simulink model "EHB_speedgoat_R2020a_V1"  (R2020a)
settings: Solver=FixedStepDiscrete  StartTime=0.0  StopTime=inf  FixedStep=0.001  RelTol=1e-3  EnableMultiTasking=on
model workspace (MAT data in the model file):
  A : Simulink.Signal (value not decoded)
  B : Simulink.Signal (value not decoded)
  C : Simulink.Signal (value not decoded)
  D : Simulink.Signal (value not decoded)
  E : Simulink.Signal (value not decoded)
  calin = [-9.96 -7.98 -5.98 -3.99 -1.994 0 1.995 3.992 5.99 7.98 9.97]
  calout = [-10 -8 -6 -4 -2 0 2 4 6 8 10]
symbols that are objects in the model workspace (value not decoded): C, D
undefined symbols (not defined in the file): Com1, none, ts_IO612
libraries: simulink x1436, xpcethercatlib x1223, yisutbxlib_utilities x256, xpcutilitieslib x156, hdlsllib x145, canmsglib x46, speedgoatlib_IO602_4 x11, speedgoatlib_IO611 x7, slrttcplib x4, CanManageLib x3, slrtlib x3, xpcseriallib x2
(part 10 of 30)

== system EHB_speedgoat_R2020a_V1/保留/TIF_06/CB1032_2/PWM ==
  Display{,1..63} (64 alike) : Display
  PCAP_DUTY_{1..32} (32 alike) : Gain
  PCAP_PER_{1..32} (32 alike) : Gain
  PWMCAP1 : Subsystem  mask(simucat_pwmcap){deviceID=0, boxNum=Box 2 (Digital Board), channel1=on, channel2=on, channel3=on, channel4=on, channel5=on, channel6=on, channel7=on, channel8=on, channel9=on, channel10=on, channel11=on, channel12=on, channel13=on, channel14=on, channel15=on, channel16=on, channel17=on, channel18=on, channel19=on, channel20=on, channel21=on, channel22=on, channel23=on, channel24=on, channel25=on, channel26=on, channel27=on, channel28=on, channel29=on, channel30=on, channel31=on, channel32=on, capMode=automatic}
      mask prompts: deviceID "Device Index:"; boxNum "Select a box:"; channel1 "1"; channel2 "2"; channel3 "3"; channel4 "4"; channel5 "5"; channel6 "6"; channel7 "7"; channel8 "8"; channel9 "9"; channel10 "10"; channel11 "11"; channel12 "12"; channel13 "13"; channel14 "14"; channel15 "15"; channel16 "16"; channel17 "17"; channel18 "18"; channel19 "19"; channel20 "20"; channel21 "21"; channel22 "22"; channel23 "23"; channel24 "24"; channel25 "25"; channel26 "26"; channel27 "27"; channel28 "28"; channel29 "29"; channel30 "30"; channel31 "31"; channel32 "32"; capMode "Cap Mode"
      mask help:
      | SimuCat系列数字板卡驱动模块。
      | 功能：PWM波捕获。通道数：32
      mask TypeOptions deviceID: 0 | 1 | 2 | 3 | 4 | 5 | 6 | 7 | 8 | 9 | 10 | 11 | 12 | 13 | 14 | 15
      mask TypeOptions boxNum: Box 1 (Digital Board) | Box 2 (Digital Board) | Box 3 (Digital Board) | Box 4 (Digital Board)
      mask TypeOptions capMode: automatic | manual
      mask DialogControl refreshButton Prompt: Refresh
      mask DialogControl refreshButton Callback: ystbx.mask.callbacks.refreshBoxList
      mask DialogControl selectChannel Prompt: Select channels:
      mask DialogControl Dummy Prompt: (Add text here)
      mask DialogControl channelSelectAll Prompt: Select All
      mask DialogControl channelSelectAll Callback: ystbx.mask.callbacks.selectAllChannels();
      mask DialogControl channelClearAll Prompt: Clear All
      mask DialogControl channelClearAll Callback: ystbx.mask.callbacks.clearAllChannels();
      mask DialogControl applyButton Prompt: Apply Modification
      mask DialogControl applyButton Callback: ystbx.mask.callbacks.maskApply();
      mask Display: disp('CB1032(Digital Board)\nPWM signal capture\nNetwork Device 0\nBox 2 (Digital Board)');port_label('output',1,'PWMCAP_DutyCycle_CH1');port_label('output',2,'PWMCAP_Period_CH1');port_label('output',3,'PWMCAP_DutyCycle_CH2');port_label('output',4,'PWMCAP_Period_CH2');port_label('output',5,'PWMCAP_DutyCycle_CH3');port_label('output',6,'PWMCAP_Period_CH3');port_label('output',7,'PWMCAP_DutyCycle_CH4');port_label('output',8,'PWMCAP_Period_CH4');port_label('output',9,'PWMCAP_DutyCycle_CH5');port_label('output',10,'PWMCAP_Period_CH5');port_label('output',11,'PWMCAP_DutyCycle_CH6');port_label('output',12,'PWMCAP_Period_CH6');port_label('output',13,'PWMCAP_DutyCycle_CH7');port_label('output',14,'PWMCAP_Period_CH7');port_label('output',15,'PWMCAP_DutyCycle_CH8');port_label('output',16,'PWMCAP_Period_CH8');port_label('output',17,'PWMCAP_DutyCycle_CH9');port_label('output',18,'PWMCAP_Period_CH9');port_label('output',19,'PWMCAP_DutyCycle_CH10');port_label('output',20,'PWMCAP_Period_CH10');port_label('output',21,'PWMCAP_DutyCycle_CH11');port_label('output',22,'PWMCAP_Period_CH11');port_label('output',23,'PWMCAP_DutyCycle_CH12');port_label('output',24,'PWMCAP_Period_CH12');port_label('output',25,'PWMCAP_DutyCycle_CH13');port_label('output',26,'PWMCAP_Period_CH13');port_label('output',27,'PWMCAP_DutyCycle_CH14');port_label('output',28,'PWMCAP_Period_CH14');port_label('output',29,'PWMCAP_DutyCycle_CH15');port_label('output',30,'PWMCAP_Period_CH15');port_label('output',31,'PWMCAP_DutyCycle_CH16');port_label('output',32,'PWMCAP_Period_CH16');port_label('output',33,'PWMCAP_DutyCycle_CH17');port_label('output',34,'PWMCAP_Period_CH17');port_label('output',35,'PWMCAP_DutyCycle_CH18');port_label('output',36,'PWMCAP_Period_CH18');port_label('output',37,'PWMCAP_DutyCycle_CH19');port_label('output',38,'PWMCAP_Period_CH19');port_label('output',39,'PWMCAP_DutyCycle_CH20');port_label('output',40,'PWMCAP_Period_CH20');port_label('output',41,'PWMCAP_DutyCycle_CH21');port_label('output',42,'PWMCAP_Period_CH21');port_label('output',43,'PWMCAP_DutyCycle_CH22');port_label('output',44,'PWMCAP_Period_CH22');port_label('output',45,'PWMCAP_DutyCycle_CH23');port_label('output',46,'PWMCAP_Period_CH23');port_label('output',47,'PWMCAP_DutyCycle_CH24');port_label('output',48,'PWMCAP_Period_CH24');port_label('output',49,'PWMCAP_DutyCycle_CH25');port_label('output',50,'PWMCAP_Period_CH25');port_label('output',51,'PWMCAP_DutyCycle_CH26');port_label('output',52,'PWMCAP_Period_CH26');port_label('output',53,'PWMCAP_DutyCycle_CH27');port_label('output',54,'PWMCAP_Period_CH27');port_label('output',55,'PWMCAP_DutyCycle_CH28');port_label('output',56,'PWMCAP_Period_CH28');port_label('output',57,'PWMCAP_DutyCycle_CH29');port_label('output',58,'PWMCAP_Period_CH29');port_label('output',59,'PWMCAP_DutyCycle_CH30');port_label('output',60,'PWMCAP_Period_CH30');port_label('output',61,'PWMCAP_DutyCycle_CH31');port_label('output',62,'PWMCAP_Period_CH31');port_label('output',63,'PWMCAP_DutyCycle_CH32');port_label('output',64,'PWMCAP_Period_CH32');
  PWMOUT : Subsystem  mask(simucat_pwmout){deviceID=0, boxNum=Box 2 (Digital Board), channel1=on, channel2=on, channel3=on, channel4=on, channel5=on, channel6=on, channel7=on, channel8=on, channel9=on, channel10=on, channel11=on, channel12=on, channel13=on, channel14=on, channel15=on, channel16=on, channel17=on, channel18=on, channel19=on, channel20=on, channel21=on, channel22=on, channel23=on, channel24=on, channel25=on, channel26=on, channel27=on, channel28=on, channel29=on, channel30=on, channel31=on, channel32=on}
      mask prompts: deviceID "Device Index:"; boxNum "Select a box:"; channel1 "1"; channel2 "2"; channel3 "3"; channel4 "4"; channel5 "5"; channel6 "6"; channel7 "7"; channel8 "8"; channel9 "9"; channel10 "10"; channel11 "11"; channel12 "12"; channel13 "13"; channel14 "14"; channel15 "15"; channel16 "16"; channel17 "17"; channel18 "18"; channel19 "19"; channel20 "20"; channel21 "21"; channel22 "22"; channel23 "23"; channel24 "24"; channel25 "25"; channel26 "26"; channel27 "27"; channel28 "28"; channel29 "29"; channel30 "30"; channel31 "31"; channel32 "32"
      mask help:
      | SimuCat系列数字板卡驱动模块。
      | 功能：PWM波输出。通道数：32
      mask TypeOptions deviceID: 0 | 1 | 2 | 3 | 4 | 5 | 6 | 7 | 8 | 9 | 10 | 11 | 12 | 13 | 14 | 15
      mask TypeOptions boxNum: Box 1 (Digital Board) | Box 2 (Digital Board) | Box 3 (Digital Board) | Box 4 (Digital Board)
      mask DialogControl refreshButton Prompt: Refresh
      mask DialogControl refreshButton Callback: ystbx.mask.callbacks.refreshBoxList
      mask DialogControl selectChannel Prompt: Select channels:
      mask DialogControl Dummy Prompt: (Add text here)
      mask DialogControl channelSelectAll Prompt: Select All
      mask DialogControl channelSelectAll Callback: ystbx.mask.callbacks.selectAllChannels();
      mask DialogControl channelClearAll Prompt: Clear All
      mask DialogControl channelClearAll Callback: ystbx.mask.callbacks.clearAllChannels();
      mask DialogControl applyButton Prompt: Apply Modification
      mask DialogControl applyButton Callback: ystbx.mask.callbacks.maskApply();
      mask Display: disp('CB1032(Digital Board)\nPWM signal output\nNetwork Device 0\nBox 2 (Digital Board)');port_label('input',1,'PWMOUT_DutyCycle_CH1');port_label('input',2,'PWMOUT_Period_CH1');port_label('input',3,'PWMOUT_DutyCycle_CH2');port_label('input',4,'PWMOUT_Period_CH2');port_label('input',5,'PWMOUT_DutyCycle_CH3');port_label('input',6,'PWMOUT_Period_CH3');port_label('input',7,'PWMOUT_DutyCycle_CH4');port_label('input',8,'PWMOUT_Period_CH4');port_label('input',9,'PWMOUT_DutyCycle_CH5');port_label('input',10,'PWMOUT_Period_CH5');port_label('input',11,'PWMOUT_DutyCycle_CH6');port_label('input',12,'PWMOUT_Period_CH6');port_label('input',13,'PWMOUT_DutyCycle_CH7');port_label('input',14,'PWMOUT_Period_CH7');port_label('input',15,'PWMOUT_DutyCycle_CH8');port_label('input',16,'PWMOUT_Period_CH8');port_label('input',17,'PWMOUT_DutyCycle_CH9');port_label('input',18,'PWMOUT_Period_CH9');port_label('input',19,'PWMOUT_DutyCycle_CH10');port_label('input',20,'PWMOUT_Period_CH10');port_label('input',21,'PWMOUT_DutyCycle_CH11');port_label('input',22,'PWMOUT_Period_CH11');port_label('input',23,'PWMOUT_DutyCycle_CH12');port_label('input',24,'PWMOUT_Period_CH12');port_label('input',25,'PWMOUT_DutyCycle_CH13');port_label('input',26,'PWMOUT_Period_CH13');port_label('input',27,'PWMOUT_DutyCycle_CH14');port_label('input',28,'PWMOUT_Period_CH14');port_label('input',29,'PWMOUT_DutyCycle_CH15');port_label('input',30,'PWMOUT_Period_CH15');port_label('input',31,'PWMOUT_DutyCycle_CH16');port_label('input',32,'PWMOUT_Period_CH16');port_label('input',33,'PWMOUT_DutyCycle_CH17');port_label('input',34,'PWMOUT_Period_CH17');port_label('input',35,'PWMOUT_DutyCycle_CH18');port_label('input',36,'PWMOUT_Period_CH18');port_label('input',37,'PWMOUT_DutyCycle_CH19');port_label('input',38,'PWMOUT_Period_CH19');port_label('input',39,'PWMOUT_DutyCycle_CH20');port_label('input',40,'PWMOUT_Period_CH20');port_label('input',41,'PWMOUT_DutyCycle_CH21');port_label('input',42,'PWMOUT_Period_CH21');port_label('input',43,'PWMOUT_DutyCycle_CH22');port_label('input',44,'PWMOUT_Period_CH22');port_label('input',45,'PWMOUT_DutyCycle_CH23');port_label('input',46,'PWMOUT_Period_CH23');port_label('input',47,'PWMOUT_DutyCycle_CH24');port_label('input',48,'PWMOUT_Period_CH24');port_label('input',49,'PWMOUT_DutyCycle_CH25');port_label('input',50,'PWMOUT_Period_CH25');port_label('input',51,'PWMOUT_DutyCycle_CH26');port_label('input',52,'PWMOUT_Period_CH26');port_label('input',53,'PWMOUT_DutyCycle_CH27');port_label('input',54,'PWMOUT_Period_CH27');port_label('input',55,'PWMOUT_DutyCycle_CH28');port_label('input',56,'PWMOUT_Period_CH28');port_label('input',57,'PWMOUT_DutyCycle_CH29');port_label('input',58,'PWMOUT_Period_CH29');port_label('input',59,'PWMOUT_DutyCycle_CH30');port_label('input',60,'PWMOUT_Period_CH30');port_label('input',61,'PWMOUT_DutyCycle_CH31');port_label('input',62,'PWMOUT_Period_CH31');port_label('input',63,'PWMOUT_DutyCycle_CH32');port_label('input',64,'PWMOUT_Period_CH32');
  PoDu_CH1 : Constant  Value=0.7
  PoDu_CH{2..32} (31 alike) : Constant  Value=0.5
  PoPe_CH{1..32} (32 alike) : Constant  Value=1/20000
  wires:
  PCAP_DUTY_30/1 -> Display58/1  "PCAP_DUTY_30"
  PCAP_DUTY_1/1 -> Display/1  "PCAP_DUTY_1"
  PCAP_DUTY_15/1 -> Display36/1  "PCAP_DUTY_15"
  PCAP_DUTY_13/1 -> Display46/1  "PCAP_DUTY_13"
  PCAP_PER_3/1 -> Display5/1  "PCAP_PER_3"
  PCAP_DUTY_19/1 -> Display20/1  "PCAP_DUTY_19"
  PCAP_DUTY_31/1 -> Display60/1  "PCAP_DUTY_31"
  PCAP_DUTY_27/1 -> Display52/1  "PCAP_DUTY_27"
  PCAP_PER_18/1 -> Display19/1  "PCAP_PER_18"
  PCAP_DUTY_32/1 -> Display62/1  "PCAP_DUTY_32"
  PCAP_DUTY_25/1 -> Display48/1  "PCAP_DUTY_25"
  PCAP_DUTY_17/1 -> Display16/1  "PCAP_DUTY_17"
  PCAP_PER_6/1 -> Display11/1  "PCAP_PER_6"
  PCAP_PER_15/1 -> Display37/1  "PCAP_PER_15"
  PCAP_PER_2/1 -> Display3/1  "PCAP_PER_2"
  PCAP_DUTY_6/1 -> Display10/1  "PCAP_DUTY_6"
  PCAP_PER_4/1 -> Display7/1  "PCAP_PER_4"
  PCAP_PER_17/1 -> Display17/1  "PCAP_PER_17"
  PCAP_DUTY_18/1 -> Display18/1  "PCAP_DUTY_18"
  PCAP_DUTY_21/1 -> Display24/1  "PCAP_DUTY_21"
  PCAP_PER_12/1 -> Display45/1  "PCAP_PER_12"
  PCAP_DUTY_10/1 -> Display40/1  "PCAP_DUTY_10"
  PCAP_PER_23/1 -> Display29/1  "PCAP_PER_23"
  PCAP_DUTY_26/1 -> Display50/1  "PCAP_DUTY_26"
  PCAP_DUTY_20/1 -> Display22/1  "PCAP_DUTY_20"
  PCAP_PER_19/1 -> Display21/1  "PCAP_PER_19"
  PCAP_DUTY_12/1 -> Display44/1  "PCAP_DUTY_12"
  PCAP_PER_29/1 -> Display57/1  "PCAP_PER_29"
  PCAP_PER_21/1 -> Display25/1  "PCAP_PER_21"
  PCAP_PER_1/1 -> Display1/1  "PCAP_PER_1"
  PCAP_DUTY_29/1 -> Display56/1  "PCAP_DUTY_29"
  PCAP_DUTY_2/1 -> Display2/1  "PCAP_DUTY_2"
  PCAP_PER_27/1 -> Display53/1  "PCAP_PER_27"
  PCAP_PER_8/1 -> Display15/1  "PCAP_PER_8"
  PCAP_PER_7/1 -> Display13/1  "PCAP_PER_7"
  PCAP_DUTY_7/1 -> Display12/1  "PCAP_DUTY_7"
  PCAP_DUTY_8/1 -> Display14/1  "PCAP_DUTY_8"
  PCAP_PER_24/1 -> Display31/1  "PCAP_PER_24"
  PCAP_PER_22/1 -> Display27/1  "PCAP_PER_22"
  PCAP_DUTY_28/1 -> Display54/1  "PCAP_DUTY_28"
  PCAP_PER_16/1 -> Display39/1  "PCAP_PER_16"
  PCAP_DUTY_11/1 -> Display42/1  "PCAP_DUTY_11"
  PCAP_DUTY_24/1 -> Display30/1  "PCAP_DUTY_24"
  PCAP_PER_30/1 -> Display59/1  "PCAP_PER_30"
  PCAP_DUTY_16/1 -> Display38/1  "PCAP_DUTY_16"
  PCAP_DUTY_4/1 -> Display6/1  "PCAP_DUTY_4"
  PCAP_DUTY_14/1 -> Display34/1  "PCAP_DUTY_14"
  PCAP_PER_10/1 -> Display41/1  "PCAP_PER_10"
  PCAP_PER_20/1 -> Display23/1  "PCAP_PER_20"
  PCAP_PER_26/1 -> Display51/1  "PCAP_PER_26"
  PCAP_PER_32/1 -> Display63/1  "PCAP_PER_32"
  PCAP_DUTY_5/1 -> Display8/1  "PCAP_DUTY_5"
  PCAP_DUTY_3/1 -> Display4/1  "PCAP_DUTY_3"
  PCAP_PER_5/1 -> Display9/1  "PCAP_PER_5"
  PCAP_DUTY_23/1 -> Display28/1  "PCAP_DUTY_23"
  PCAP_DUTY_22/1 -> Display26/1  "PCAP_DUTY_22"
  PCAP_DUTY_9/1 -> Display32/1  "PCAP_DUTY_9"
  PCAP_PER_25/1 -> Display49/1  "PCAP_PER_25"
  PCAP_PER_13/1 -> Display47/1  "PCAP_PER_13"
  PCAP_PER_9/1 -> Display33/1  "PCAP_PER_9"
  PCAP_PER_28/1 -> Display55/1  "PCAP_PER_28"
  PCAP_PER_31/1 -> Display61/1  "PCAP_PER_31"
  PCAP_PER_11/1 -> Display43/1  "PCAP_PER_11"
  PCAP_PER_14/1 -> Display35/1  "PCAP_PER_14"
  PWMCAP1/2(PWMCAP_Period_CH1) -> PCAP_PER_1/1
  PWMCAP1/4(PWMCAP_Period_CH2) -> PCAP_PER_2/1
  PWMCAP1/6(PWMCAP_Period_CH3) -> PCAP_PER_3/1
  PWMCAP1/8(PWMCAP_Period_CH4) -> PCAP_PER_4/1
  PWMCAP1/10(PWMCAP_Period_CH5) -> PCAP_PER_5/1
  PWMCAP1/12(PWMCAP_Period_CH6) -> PCAP_PER_6/1
  PWMCAP1/14(PWMCAP_Period_CH7) -> PCAP_PER_7/1
  PWMCAP1/16(PWMCAP_Period_CH8) -> PCAP_PER_8/1
  PWMCAP1/18(PWMCAP_Period_CH9) -> PCAP_PER_9/1
  PWMCAP1/20(PWMCAP_Period_CH10) -> PCAP_PER_10/1
  PWMCAP1/22(PWMCAP_Period_CH11) -> PCAP_PER_11/1
  PWMCAP1/24(PWMCAP_Period_CH12) -> PCAP_PER_12/1
  PWMCAP1/26(PWMCAP_Period_CH13) -> PCAP_PER_13/1
  PWMCAP1/28(PWMCAP_Period_CH14) -> PCAP_PER_14/1
  PWMCAP1/30(PWMCAP_Period_CH15) -> PCAP_PER_15/1
  PWMCAP1/32(PWMCAP_Period_CH16) -> PCAP_PER_16/1
  PWMCAP1/34(PWMCAP_Period_CH17) -> PCAP_PER_17/1
  PWMCAP1/36(PWMCAP_Period_CH18) -> PCAP_PER_18/1
  PWMCAP1/38(PWMCAP_Period_CH19) -> PCAP_PER_19/1
  PWMCAP1/40(PWMCAP_Period_CH20) -> PCAP_PER_20/1
  PWMCAP1/42(PWMCAP_Period_CH21) -> PCAP_PER_21/1
  PWMCAP1/44(PWMCAP_Period_CH22) -> PCAP_PER_22/1
  PWMCAP1/46(PWMCAP_Period_CH23) -> PCAP_PER_23/1
  PWMCAP1/48(PWMCAP_Period_CH24) -> PCAP_PER_24/1
  PWMCAP1/50(PWMCAP_Period_CH25) -> PCAP_PER_25/1
  PWMCAP1/52(PWMCAP_Period_CH26) -> PCAP_PER_26/1
  PWMCAP1/54(PWMCAP_Period_CH27) -> PCAP_PER_27/1
  PWMCAP1/56(PWMCAP_Period_CH28) -> PCAP_PER_28/1
  PWMCAP1/58(PWMCAP_Period_CH29) -> PCAP_PER_29/1
  PWMCAP1/60(PWMCAP_Period_CH30) -> PCAP_PER_30/1
  PWMCAP1/62(PWMCAP_Period_CH31) -> PCAP_PER_31/1
  PWMCAP1/64(PWMCAP_Period_CH32) -> PCAP_PER_32/1
  PWMCAP1/1(PWMCAP_DutyCycle_CH1) -> PCAP_DUTY_1/1
  PWMCAP1/3(PWMCAP_DutyCycle_CH2) -> PCAP_DUTY_2/1
  PWMCAP1/5(PWMCAP_DutyCycle_CH3) -> PCAP_DUTY_3/1
  PWMCAP1/7(PWMCAP_DutyCycle_CH4) -> PCAP_DUTY_4/1
  PWMCAP1/9(PWMCAP_DutyCycle_CH5) -> PCAP_DUTY_5/1
  PWMCAP1/11(PWMCAP_DutyCycle_CH6) -> PCAP_DUTY_6/1
  PWMCAP1/13(PWMCAP_DutyCycle_CH7) -> PCAP_DUTY_7/1
  PWMCAP1/15(PWMCAP_DutyCycle_CH8) -> PCAP_DUTY_8/1
  PWMCAP1/17(PWMCAP_DutyCycle_CH9) -> PCAP_DUTY_9/1
  PWMCAP1/19(PWMCAP_DutyCycle_CH10) -> PCAP_DUTY_10/1
  PWMCAP1/21(PWMCAP_DutyCycle_CH11) -> PCAP_DUTY_11/1
  PWMCAP1/23(PWMCAP_DutyCycle_CH12) -> PCAP_DUTY_12/1
  PWMCAP1/25(PWMCAP_DutyCycle_CH13) -> PCAP_DUTY_13/1
  PWMCAP1/27(PWMCAP_DutyCycle_CH14) -> PCAP_DUTY_14/1
  PWMCAP1/29(PWMCAP_DutyCycle_CH15) -> PCAP_DUTY_15/1
  PWMCAP1/31(PWMCAP_DutyCycle_CH16) -> PCAP_DUTY_16/1
  PWMCAP1/33(PWMCAP_DutyCycle_CH17) -> PCAP_DUTY_17/1
  PWMCAP1/35(PWMCAP_DutyCycle_CH18) -> PCAP_DUTY_18/1
  PWMCAP1/37(PWMCAP_DutyCycle_CH19) -> PCAP_DUTY_19/1
  PWMCAP1/39(PWMCAP_DutyCycle_CH20) -> PCAP_DUTY_20/1
  PWMCAP1/41(PWMCAP_DutyCycle_CH21) -> PCAP_DUTY_21/1
  PWMCAP1/43(PWMCAP_DutyCycle_CH22) -> PCAP_DUTY_22/1
  PWMCAP1/45(PWMCAP_DutyCycle_CH23) -> PCAP_DUTY_23/1
  PWMCAP1/47(PWMCAP_DutyCycle_CH24) -> PCAP_DUTY_24/1
  PWMCAP1/49(PWMCAP_DutyCycle_CH25) -> PCAP_DUTY_25/1
  PWMCAP1/51(PWMCAP_DutyCycle_CH26) -> PCAP_DUTY_26/1
  PWMCAP1/53(PWMCAP_DutyCycle_CH27) -> PCAP_DUTY_27/1
  PWMCAP1/55(PWMCAP_DutyCycle_CH28) -> PCAP_DUTY_28/1
  PWMCAP1/57(PWMCAP_DutyCycle_CH29) -> PCAP_DUTY_29/1
  PWMCAP1/59(PWMCAP_DutyCycle_CH30) -> PCAP_DUTY_30/1
  PWMCAP1/61(PWMCAP_DutyCycle_CH31) -> PCAP_DUTY_31/1
  PWMCAP1/63(PWMCAP_DutyCycle_CH32) -> PCAP_DUTY_32/1
  PoDu_CH19/1 -> PWMOUT/37(PWMOUT_DutyCycle_CH19)  "PoDu_CH19"
  PoPe_CH19/1 -> PWMOUT/38(PWMOUT_Period_CH19)  "PoPe_CH19"
  PoDu_CH20/1 -> PWMOUT/39(PWMOUT_DutyCycle_CH20)  "PoDu_CH20"
  PoPe_CH21/1 -> PWMOUT/42(PWMOUT_Period_CH21)  "PoPe_CH21"
  PoDu_CH22/1 -> PWMOUT/43(PWMOUT_DutyCycle_CH22)  "PoDu_CH22"
  PoDu_CH1/1 -> PWMOUT/1(PWMOUT_DutyCycle_CH1)  "PoDu_CH17"
  PoPe_CH1/1 -> PWMOUT/2(PWMOUT_Period_CH1)  "PoPe_CH17"
  PoDu_CH2/1 -> PWMOUT/3(PWMOUT_DutyCycle_CH2)  "PoDu_CH18"
  PoPe_CH2/1 -> PWMOUT/4(PWMOUT_Period_CH2)  "PoPe_CH18"
  PoDu_CH3/1 -> PWMOUT/5(PWMOUT_DutyCycle_CH3)  "PoDu_CH19"
  PoPe_CH3/1 -> PWMOUT/6(PWMOUT_Period_CH3)  "PoPe_CH19"
  PoDu_CH4/1 -> PWMOUT/7(PWMOUT_DutyCycle_CH4)  "PoDu_CH20"
  PoPe_CH4/1 -> PWMOUT/8(PWMOUT_Period_CH4)  "PoPe_CH20"
  PoDu_CH5/1 -> PWMOUT/9(PWMOUT_DutyCycle_CH5)  "PoDu_CH21"
  PoPe_CH5/1 -> PWMOUT/10(PWMOUT_Period_CH5)  "PoPe_CH21"
  PoDu_CH6/1 -> PWMOUT/11(PWMOUT_DutyCycle_CH6)  "PoDu_CH22"
  PoPe_CH6/1 -> PWMOUT/12(PWMOUT_Period_CH6)  "PoPe_CH22"
  PoDu_CH7/1 -> PWMOUT/13(PWMOUT_DutyCycle_CH7)  "PoDu_CH23"
  PoPe_CH7/1 -> PWMOUT/14(PWMOUT_Period_CH7)  "PoPe_CH23"
  PoDu_CH8/1 -> PWMOUT/15(PWMOUT_DutyCycle_CH8)  "PoDu_CH24"
  PoPe_CH8/1 -> PWMOUT/16(PWMOUT_Period_CH8)  "PoPe_CH24"
  PoDu_CH9/1 -> PWMOUT/17(PWMOUT_DutyCycle_CH9)  "PoDu_CH25"
  PoPe_CH9/1 -> PWMOUT/18(PWMOUT_Period_CH9)  "PoPe_CH25"
  PoDu_CH10/1 -> PWMOUT/19(PWMOUT_DutyCycle_CH10)  "PoDu_CH26"
  PoPe_CH10/1 -> PWMOUT/20(PWMOUT_Period_CH10)  "PoPe_CH26"
  PoDu_CH11/1 -> PWMOUT/21(PWMOUT_DutyCycle_CH11)  "PoDu_CH27"
  PoPe_CH11/1 -> PWMOUT/22(PWMOUT_Period_CH11)  "PoPe_CH27"
  PoDu_CH12/1 -> PWMOUT/23(PWMOUT_DutyCycle_CH12)  "PoDu_CH28"
  PoPe_CH12/1 -> PWMOUT/24(PWMOUT_Period_CH12)  "PoPe_CH28"
  PoDu_CH13/1 -> PWMOUT/25(PWMOUT_DutyCycle_CH13)  "PoDu_CH29"
  PoPe_CH13/1 -> PWMOUT/26(PWMOUT_Period_CH13)  "PoPe_CH29"
  PoDu_CH14/1 -> PWMOUT/27(PWMOUT_DutyCycle_CH14)  "PoDu_CH30"
  PoPe_CH14/1 -> PWMOUT/28(PWMOUT_Period_CH14)  "PoPe_CH30"
  PoDu_CH15/1 -> PWMOUT/29(PWMOUT_DutyCycle_CH15)  "PoDu_CH31"
  PoPe_CH15/1 -> PWMOUT/30(PWMOUT_Period_CH15)  "PoPe_CH31"
  PoDu_CH16/1 -> PWMOUT/31(PWMOUT_DutyCycle_CH16)  "PoDu_CH32"
  PoPe_CH16/1 -> PWMOUT/32(PWMOUT_Period_CH16)  "PoPe_CH32"
  PoDu_CH17/1 -> PWMOUT/33(PWMOUT_DutyCycle_CH17)  "PoDu_CH17"
  PoPe_CH17/1 -> PWMOUT/34(PWMOUT_Period_CH17)  "PoPe_CH17"
  PoDu_CH18/1 -> PWMOUT/35(PWMOUT_DutyCycle_CH18)  "PoDu_CH18"
  PoPe_CH18/1 -> PWMOUT/36(PWMOUT_Period_CH18)  "PoPe_CH18"
  PoPe_CH20/1 -> PWMOUT/40(PWMOUT_Period_CH20)  "PoPe_CH20"
  PoDu_CH21/1 -> PWMOUT/41(PWMOUT_DutyCycle_CH21)  "PoDu_CH21"
  PoPe_CH22/1 -> PWMOUT/44(PWMOUT_Period_CH22)  "PoPe_CH22"
  PoDu_CH23/1 -> PWMOUT/45(PWMOUT_DutyCycle_CH23)  "PoDu_CH23"
  PoPe_CH23/1 -> PWMOUT/46(PWMOUT_Period_CH23)  "PoPe_CH23"
  PoDu_CH24/1 -> PWMOUT/47(PWMOUT_DutyCycle_CH24)  "PoDu_CH24"
  PoPe_CH24/1 -> PWMOUT/48(PWMOUT_Period_CH24)  "PoPe_CH24"
  PoDu_CH25/1 -> PWMOUT/49(PWMOUT_DutyCycle_CH25)  "PoDu_CH25"
  PoPe_CH25/1 -> PWMOUT/50(PWMOUT_Period_CH25)  "PoPe_CH25"
  PoDu_CH26/1 -> PWMOUT/51(PWMOUT_DutyCycle_CH26)  "PoDu_CH26"
  PoPe_CH26/1 -> PWMOUT/52(PWMOUT_Period_CH26)  "PoPe_CH26"
  PoDu_CH27/1 -> PWMOUT/53(PWMOUT_DutyCycle_CH27)  "PoDu_CH27"
  PoPe_CH27/1 -> PWMOUT/54(PWMOUT_Period_CH27)  "PoPe_CH27"
  PoDu_CH28/1 -> PWMOUT/55(PWMOUT_DutyCycle_CH28)  "PoDu_CH28"
  PoPe_CH28/1 -> PWMOUT/56(PWMOUT_Period_CH28)  "PoPe_CH28"
  PoDu_CH29/1 -> PWMOUT/57(PWMOUT_DutyCycle_CH29)  "PoDu_CH29"
  PoPe_CH29/1 -> PWMOUT/58(PWMOUT_Period_CH29)  "PoPe_CH29"
  PoDu_CH30/1 -> PWMOUT/59(PWMOUT_DutyCycle_CH30)  "PoDu_CH30"
  PoPe_CH30/1 -> PWMOUT/60(PWMOUT_Period_CH30)  "PoPe_CH30"
  PoDu_CH31/1 -> PWMOUT/61(PWMOUT_DutyCycle_CH31)  "PoDu_CH31"
  PoPe_CH31/1 -> PWMOUT/62(PWMOUT_Period_CH31)  "PoPe_CH31"
  PoDu_CH32/1 -> PWMOUT/63(PWMOUT_DutyCycle_CH32)  "PoDu_CH32"
  PoPe_CH32/1 -> PWMOUT/64(PWMOUT_Period_CH32)  "PoPe_CH32"

== system EHB_speedgoat_R2020a_V1/保留/TIF_06/YS4020_M_1/YS4020_M ==
  FIU_SetCH1 : Inport
  FIU_SetCH2 : Inport  Port=2
  FIU_SetCH3 : Inport  Port=3
  FIU_SetCH4 : Inport  Port=4
  FIU_SetCH5 : Inport  Port=5
  FIU_SetCH6 : Inport  Port=6
  FIU_SetCH7 : Inport  Port=7
  FIU_SetCH8 : Inport  Port=8
  FIU_SetCH9 : Inport  Port=9
  FIU_SetCH10 : Inport  Port=10
  FIU_SetCH11 : Inport  Port=11
  FIU_SetCH12 : Inport  Port=12
  FIU_SetCH13 : Inport  Port=13
  FIU_SetCH14 : Inport  Port=14
  FIU_SetCH15 : Inport  Port=15
  FIU_SetCH16 : Inport  Port=16
  FIU_SetCH17 : Inport  Port=17
  FIU_SetCH18 : Inport  Port=18
  FIU_SetCH19 : Inport  Port=19
  FIU_SetCH20 : Inport  Port=20
  PassWord : Inport  Port=21
  YS4020_M_Slot : Inport  Port=22
  Bus Creator : BusCreator  Inputs=12
  Bus Creator1 : BusCreator  Inputs=12
  Demux : Demux  Outputs=10
  Demux1 : Demux  Outputs=10
  FIU_CH1 : Subsystem
  FIU_CH10 : Subsystem
  FIU_CH11 : Subsystem
  FIU_CH12 : Subsystem
  FIU_CH13 : Subsystem
  FIU_CH14 : Subsystem
  FIU_CH15 : Subsystem
  FIU_CH16 : Subsystem
  FIU_CH17 : Subsystem
  FIU_CH18 : Subsystem
  FIU_CH19 : Subsystem
  FIU_CH2 : Subsystem
  FIU_CH20 : Subsystem
  FIU_CH3 : Subsystem
  FIU_CH4 : Subsystem
  FIU_CH5 : Subsystem
  FIU_CH6 : Subsystem
  FIU_CH7 : Subsystem
  FIU_CH8 : Subsystem
  FIU_CH9 : Subsystem
  FIU_MsgSend : Subsystem
  FIU_MsgSend1 : Subsystem
  Mux : Mux  Inputs=10
  Mux1 : Mux  Inputs=10
  YS4020_M_Ctrl_Trigger : Subsystem
  YS4020_M_Ctrl_Trigger1 : Subsystem
  tag scope: YS4020_M_1_1=global, YS4020_M_1_2=global
  wires:
  FIU_SetCH1/1 -> Mux/1
  FIU_SetCH2/1 -> Mux/2
  FIU_SetCH3/1 -> Mux/3
  FIU_SetCH4/1 -> Mux/4
  FIU_SetCH5/1 -> Mux/5
  FIU_SetCH6/1 -> Mux/6
  FIU_SetCH7/1 -> Mux/7
  FIU_SetCH8/1 -> Mux/8
  FIU_SetCH9/1 -> Mux/9
  FIU_SetCH10/1 -> Mux/10
  FIU_SetCH11/1 -> Mux1/1
  FIU_SetCH12/1 -> Mux1/2
  FIU_SetCH13/1 -> Mux1/3
  FIU_SetCH14/1 -> Mux1/4
  FIU_SetCH15/1 -> Mux1/5
  FIU_SetCH16/1 -> Mux1/6
  FIU_SetCH17/1 -> Mux1/7
  FIU_SetCH18/1 -> Mux1/8
  FIU_SetCH19/1 -> Mux1/9
  FIU_SetCH20/1 -> Mux1/10
  Mux/1 -> Demux/1, [CH1_10]
  Demux/1 -> FIU_CH1/1(FIU_SetCH1)
  YS4020_M_Ctrl_Trigger/1(YS4020_M_CtrlTrigger) -> FIU_MsgSend/Enable  "Trigger"
  Demux/2 -> FIU_CH2/1(FIU_SetCH2)
  Demux/3 -> FIU_CH3/1(FIU_SetCH3)
  Demux/4 -> FIU_CH4/1(FIU_SetCH4)
  Demux/5 -> FIU_CH5/1(FIU_SetCH5)
  Demux/6 -> FIU_CH6/1(FIU_SetCH6)
  Demux/7 -> FIU_CH7/1(FIU_SetCH7)
  Demux/8 -> FIU_CH8/1(FIU_SetCH8)
  Demux/9 -> FIU_CH9/1(FIU_SetCH9)
  Demux/10 -> FIU_CH10/1(FIU_SetCH10)
  FIU_CH1/1(CH1_Out) -> Bus Creator/3  "CH1_Out"
  FIU_CH2/1(CH2_Out) -> Bus Creator/4  "CH2_Out"
  FIU_CH3/1(CH3_Out) -> Bus Creator/5  "CH3_Out"
  FIU_CH4/1(CH4_Out) -> Bus Creator/6  "CH4_Out"
  FIU_CH5/1(CH5_Out) -> Bus Creator/7  "CH5_Out"
  FIU_CH6/1(CH6_Out) -> Bus Creator/8  "CH6_Out"
  FIU_CH7/1(CH7_Out) -> Bus Creator/9  "CH7_Out"
  FIU_CH8/1(CH8_Out) -> Bus Creator/10  "CH8_Out"
  FIU_CH9/1(CH9_Out) -> Bus Creator/11  "CH9_Out"
  FIU_CH10/1(CH10_Out) -> Bus Creator/12  "CH10_Out"
  [CH1_10] -> YS4020_M_Ctrl_Trigger/1(CH1_10)
  Bus Creator/1 -> FIU_MsgSend/1(YS4020_M)  "YS4020_M"
  YS4020_M_Slot/1 -> [Slot]  "YS4020_M_Slot"
  PassWord/1 -> [PassWord]  "PassWord"
  [PassWord] -> Bus Creator/1
  [Slot] -> Bus Creator/2
  [Slot] -> Bus Creator1/2
  [PassWord] -> Bus Creator1/1
  Bus Creator1/1 -> FIU_MsgSend1/1(YS4020_M)  "YS4020_M"
  [CH11_20] -> YS4020_M_Ctrl_Trigger1/1(CH11_20)
  FIU_CH12/1(CH10_Out) -> Bus Creator1/12  "CH10_Out"
  FIU_CH20/1(CH9_Out) -> Bus Creator1/11  "CH9_Out"
  FIU_CH19/1(CH8_Out) -> Bus Creator1/10  "CH8_Out"
  FIU_CH18/1(CH7_Out) -> Bus Creator1/9  "CH7_Out"
  FIU_CH17/1(CH6_Out) -> Bus Creator1/8  "CH6_Out"
  FIU_CH16/1(CH5_Out) -> Bus Creator1/7  "CH5_Out"
  FIU_CH15/1(CH4_Out) -> Bus Creator1/6  "CH4_Out"
  FIU_CH14/1(CH3_Out) -> Bus Creator1/5  "CH3_Out"
  FIU_CH13/1(CH2_Out) -> Bus Creator1/4  "CH2_Out"
  FIU_CH11/1(CH1_Out) -> Bus Creator1/3  "CH1_Out"
  Demux1/10 -> FIU_CH12/1(FIU_SetCH10)
  Demux1/9 -> FIU_CH20/1(FIU_SetCH9)
  Demux1/8 -> FIU_CH19/1(FIU_SetCH8)
  Demux1/7 -> FIU_CH18/1(FIU_SetCH7)
  Demux1/6 -> FIU_CH17/1(FIU_SetCH6)
  Demux1/5 -> FIU_CH16/1(FIU_SetCH5)
  Demux1/4 -> FIU_CH15/1(FIU_SetCH4)
  Demux1/3 -> FIU_CH14/1(FIU_SetCH3)
  Demux1/2 -> FIU_CH13/1(FIU_SetCH2)
  YS4020_M_Ctrl_Trigger1/1(YS4020_M_CtrlTrigger) -> FIU_MsgSend1/Enable  "Trigger"
  Demux1/1 -> FIU_CH11/1(FIU_SetCH1)
  Mux1/1 -> Demux1/1, [CH11_20]
  FIU_MsgSend/1(Output) -> [YS4020_M_1_1]
  FIU_MsgSend1/1(Output) -> [YS4020_M_1_2]

== system EHB_speedgoat_R2020a_V1/保留/YS4008/YS4008_M_1/YS4008_M ==
  PassWord : Inport
  FIU_SetCH1 : Inport  Port=2
  FIU_SetCH2 : Inport  Port=3
  FIU_SetCH3 : Inport  Port=4
  FIU_SetCH4 : Inport  Port=5
  FIU_SetCH5 : Inport  Port=6
  FIU_SetCH6 : Inport  Port=7
  FIU_SetCH7 : Inport  Port=8
  FIU_SetCH8 : Inport  Port=9
  Rack : Inport  Port=10
  Slot : Inport  Port=11
  Bus Creator : BusCreator  Inputs=11
  Bus Creator1 : BusCreator  Inputs=8
  Bus Selector : BusSelector  OutputSignals=FIU_SetCH1,FIU_SetCH2,FIU_SetCH3,FIU_SetCH4,FIU_SetCH5,FIU_SetCH6,FIU_SetCH7,FIU_SetCH8
  FIU_CH1 : Subsystem
  FIU_CH2 : Subsystem
  FIU_CH3 : Subsystem
  FIU_CH4 : Subsystem
  FIU_CH5 : Subsystem
  FIU_CH6 : Subsystem
  FIU_CH7 : Subsystem
  FIU_CH8 : Subsystem
  FIU_MsgSend : Subsystem
  YS4008_M_Ctrl_Trigger : Subsystem
  Output : Outport
  wires:
  Bus Creator/1 -> FIU_MsgSend/1(YS4008_M)  "YS4008_M"
  YS4008_M_Ctrl_Trigger/1(YS4008_M_CtrlTrigger) -> FIU_MsgSend/Enable  "Trigger"
  FIU_CH1/1(CH1_Out) -> Bus Creator/2  "CH1_Out"
  FIU_CH2/1(CH2_Out) -> Bus Creator/3  "CH2_Out"
  FIU_CH3/1(CH3_Out) -> Bus Creator/4  "CH3_Out"
  FIU_CH4/1(CH4_Out) -> Bus Creator/5  "CH4_Out"
  FIU_CH5/1(CH5_Out) -> Bus Creator/6  "CH5_Out"
  FIU_CH6/1(CH6_Out) -> Bus Creator/7  "CH6_Out"
  FIU_CH7/1(CH7_Out) -> Bus Creator/8  "CH7_Out"
  FIU_CH8/1(CH8_Out) -> Bus Creator/9  "CH8_Out"
  PassWord/1 -> Bus Creator/1  "PassWord"
  FIU_SetCH1/1 -> Bus Creator1/1  "FIU_SetCH1"
  FIU_SetCH2/1 -> Bus Creator1/2  "FIU_SetCH2"
  FIU_SetCH3/1 -> Bus Creator1/3  "FIU_SetCH3"
  FIU_SetCH7/1 -> Bus Creator1/7  "FIU_SetCH7"
  FIU_SetCH8/1 -> Bus Creator1/8  "FIU_SetCH8"
  FIU_SetCH4/1 -> Bus Creator1/4  "FIU_SetCH4"
  FIU_SetCH5/1 -> Bus Creator1/5  "FIU_SetCH5"
  FIU_SetCH6/1 -> Bus Creator1/6  "FIU_SetCH6"
  Bus Creator1/1 -> [FIU_Set], Bus Selector/1
  [FIU_Set] -> YS4008_M_Ctrl_Trigger/1(YS4008_M)
  Bus Selector/1 -> FIU_CH1/1(FIU_SetCH1)  "<FIU_SetCH1>"
  Bus Selector/2 -> FIU_CH2/1(FIU_SetCH2)  "<FIU_SetCH2>"
  Bus Selector/3 -> FIU_CH3/1(FIU_SetCH3)  "<FIU_SetCH3>"
  Bus Selector/4 -> FIU_CH4/1(FIU_SetCH4)  "<FIU_SetCH4>"
  Bus Selector/5 -> FIU_CH5/1(FIU_SetCH5)  "<FIU_SetCH5>"
  Bus Selector/6 -> FIU_CH6/1(FIU_SetCH6)  "<FIU_SetCH6>"
  Bus Selector/7 -> FIU_CH7/1(FIU_SetCH7)  "<FIU_SetCH7>"
  Bus Selector/8 -> FIU_CH8/1(FIU_SetCH8)  "<FIU_SetCH8>"
  Rack/1 -> Bus Creator/10  "Rack"
  Slot/1 -> Bus Creator/11  "Slot"
  FIU_MsgSend/1(Output) -> Output/1

== system EHB_speedgoat_R2020a_V1/保留/YS4008/YS4008_M_2/YS4008_M ==
  PassWord : Inport
  FIU_SetCH1 : Inport  Port=2
  FIU_SetCH2 : Inport  Port=3
  FIU_SetCH3 : Inport  Port=4
  FIU_SetCH4 : Inport  Port=5
  FIU_SetCH5 : Inport  Port=6
  FIU_SetCH6 : Inport  Port=7
  FIU_SetCH7 : Inport  Port=8
  FIU_SetCH8 : Inport  Port=9
  Rack : Inport  Port=10
  Slot : Inport  Port=11
  Bus Creator : BusCreator  Inputs=11
  Bus Creator1 : BusCreator  Inputs=8
  Bus Selector : BusSelector  OutputSignals=FIU_SetCH1,FIU_SetCH2,FIU_SetCH3,FIU_SetCH4,FIU_SetCH5,FIU_SetCH6,FIU_SetCH7,FIU_SetCH8
  FIU_CH1 : Subsystem
  FIU_CH2 : Subsystem
  FIU_CH3 : Subsystem
  FIU_CH4 : Subsystem
  FIU_CH5 : Subsystem
  FIU_CH6 : Subsystem
  FIU_CH7 : Subsystem
  FIU_CH8 : Subsystem
  FIU_MsgSend : Subsystem
  YS4008_M_Ctrl_Trigger : Subsystem
  Output : Outport
  wires:
  Bus Creator/1 -> FIU_MsgSend/1(YS4008_M)  "YS4008_M"
  YS4008_M_Ctrl_Trigger/1(YS4008_M_CtrlTrigger) -> FIU_MsgSend/Enable  "Trigger"
  FIU_CH1/1(CH1_Out) -> Bus Creator/2  "CH1_Out"
  FIU_CH2/1(CH2_Out) -> Bus Creator/3  "CH2_Out"
  FIU_CH3/1(CH3_Out) -> Bus Creator/4  "CH3_Out"
  FIU_CH4/1(CH4_Out) -> Bus Creator/5  "CH4_Out"
  FIU_CH5/1(CH5_Out) -> Bus Creator/6  "CH5_Out"
  FIU_CH6/1(CH6_Out) -> Bus Creator/7  "CH6_Out"
  FIU_CH7/1(CH7_Out) -> Bus Creator/8  "CH7_Out"
  FIU_CH8/1(CH8_Out) -> Bus Creator/9  "CH8_Out"
  PassWord/1 -> Bus Creator/1  "PassWord"
  FIU_SetCH1/1 -> Bus Creator1/1  "FIU_SetCH1"
  FIU_SetCH2/1 -> Bus Creator1/2  "FIU_SetCH2"
  FIU_SetCH3/1 -> Bus Creator1/3  "FIU_SetCH3"
  FIU_SetCH7/1 -> Bus Creator1/7  "FIU_SetCH7"
  FIU_SetCH8/1 -> Bus Creator1/8  "FIU_SetCH8"
  FIU_SetCH4/1 -> Bus Creator1/4  "FIU_SetCH4"
  FIU_SetCH5/1 -> Bus Creator1/5  "FIU_SetCH5"
  FIU_SetCH6/1 -> Bus Creator1/6  "FIU_SetCH6"
  Bus Creator1/1 -> [FIU_Set], Bus Selector/1
  [FIU_Set] -> YS4008_M_Ctrl_Trigger/1(YS4008_M)
  Bus Selector/1 -> FIU_CH1/1(FIU_SetCH1)  "<FIU_SetCH1>"
  Bus Selector/2 -> FIU_CH2/1(FIU_SetCH2)  "<FIU_SetCH2>"
  Bus Selector/3 -> FIU_CH3/1(FIU_SetCH3)  "<FIU_SetCH3>"
  Bus Selector/4 -> FIU_CH4/1(FIU_SetCH4)  "<FIU_SetCH4>"
  Bus Selector/5 -> FIU_CH5/1(FIU_SetCH5)  "<FIU_SetCH5>"
  Bus Selector/6 -> FIU_CH6/1(FIU_SetCH6)  "<FIU_SetCH6>"
  Bus Selector/7 -> FIU_CH7/1(FIU_SetCH7)  "<FIU_SetCH7>"
  Bus Selector/8 -> FIU_CH8/1(FIU_SetCH8)  "<FIU_SetCH8>"
  Rack/1 -> Bus Creator/10  "Rack"
  Slot/1 -> Bus Creator/11  "Slot"
  FIU_MsgSend/1(Output) -> Output/1

== system EHB_speedgoat_R2020a_V1/保留/YS4008/YS4008_M_3/YS4008_M ==
  PassWord : Inport
  FIU_SetCH1 : Inport  Port=2
  FIU_SetCH2 : Inport  Port=3
  FIU_SetCH3 : Inport  Port=4
  FIU_SetCH4 : Inport  Port=5
  FIU_SetCH5 : Inport  Port=6
  FIU_SetCH6 : Inport  Port=7
  FIU_SetCH7 : Inport  Port=8
  FIU_SetCH8 : Inport  Port=9
  Rack : Inport  Port=10
  Slot : Inport  Port=11
  Bus Creator : BusCreator  Inputs=11
  Bus Creator1 : BusCreator  Inputs=8
  Bus Selector : BusSelector  OutputSignals=FIU_SetCH1,FIU_SetCH2,FIU_SetCH3,FIU_SetCH4,FIU_SetCH5,FIU_SetCH6,FIU_SetCH7,FIU_SetCH8
  FIU_CH1 : Subsystem
  FIU_CH2 : Subsystem
  FIU_CH3 : Subsystem
  FIU_CH4 : Subsystem
  FIU_CH5 : Subsystem
  FIU_CH6 : Subsystem
  FIU_CH7 : Subsystem
  FIU_CH8 : Subsystem
  FIU_MsgSend : Subsystem
  YS4008_M_Ctrl_Trigger : Subsystem
  Output : Outport
  wires:
  Bus Creator/1 -> FIU_MsgSend/1(YS4008_M)  "YS4008_M"
  YS4008_M_Ctrl_Trigger/1(YS4008_M_CtrlTrigger) -> FIU_MsgSend/Enable  "Trigger"
  FIU_CH1/1(CH1_Out) -> Bus Creator/2  "CH1_Out"
  FIU_CH2/1(CH2_Out) -> Bus Creator/3  "CH2_Out"
  FIU_CH3/1(CH3_Out) -> Bus Creator/4  "CH3_Out"
  FIU_CH4/1(CH4_Out) -> Bus Creator/5  "CH4_Out"
  FIU_CH5/1(CH5_Out) -> Bus Creator/6  "CH5_Out"
  FIU_CH6/1(CH6_Out) -> Bus Creator/7  "CH6_Out"
  FIU_CH7/1(CH7_Out) -> Bus Creator/8  "CH7_Out"
  FIU_CH8/1(CH8_Out) -> Bus Creator/9  "CH8_Out"
  PassWord/1 -> Bus Creator/1  "PassWord"
  FIU_SetCH1/1 -> Bus Creator1/1  "FIU_SetCH1"
  FIU_SetCH2/1 -> Bus Creator1/2  "FIU_SetCH2"
  FIU_SetCH3/1 -> Bus Creator1/3  "FIU_SetCH3"
  FIU_SetCH7/1 -> Bus Creator1/7  "FIU_SetCH7"
  FIU_SetCH8/1 -> Bus Creator1/8  "FIU_SetCH8"
  FIU_SetCH4/1 -> Bus Creator1/4  "FIU_SetCH4"
  FIU_SetCH5/1 -> Bus Creator1/5  "FIU_SetCH5"
  FIU_SetCH6/1 -> Bus Creator1/6  "FIU_SetCH6"
  Bus Creator1/1 -> [FIU_Set], Bus Selector/1
  [FIU_Set] -> YS4008_M_Ctrl_Trigger/1(YS4008_M)
  Bus Selector/1 -> FIU_CH1/1(FIU_SetCH1)  "<FIU_SetCH1>"
  Bus Selector/2 -> FIU_CH2/1(FIU_SetCH2)  "<FIU_SetCH2>"
  Bus Selector/3 -> FIU_CH3/1(FIU_SetCH3)  "<FIU_SetCH3>"
  Bus Selector/4 -> FIU_CH4/1(FIU_SetCH4)  "<FIU_SetCH4>"
  Bus Selector/5 -> FIU_CH5/1(FIU_SetCH5)  "<FIU_SetCH5>"
  Bus Selector/6 -> FIU_CH6/1(FIU_SetCH6)  "<FIU_SetCH6>"
  Bus Selector/7 -> FIU_CH7/1(FIU_SetCH7)  "<FIU_SetCH7>"
  Bus Selector/8 -> FIU_CH8/1(FIU_SetCH8)  "<FIU_SetCH8>"
  Rack/1 -> Bus Creator/10  "Rack"
  Slot/1 -> Bus Creator/11  "Slot"
  FIU_MsgSend/1(Output) -> Output/1

== system EHB_speedgoat_R2020a_V1/保留/YS4008/YS4008_M_4/YS4008_M1 ==
  PassWord : Inport
  FIU_SetCH1 : Inport  Port=2
  FIU_SetCH2 : Inport  Port=3
  FIU_SetCH3 : Inport  Port=4
  FIU_SetCH4 : Inport  Port=5
  FIU_SetCH5 : Inport  Port=6
  FIU_SetCH6 : Inport  Port=7
  FIU_SetCH7 : Inport  Port=8
  FIU_SetCH8 : Inport  Port=9
  Rack : Inport  Port=10
  Slot : Inport  Port=11
  Bus Creator : BusCreator  Inputs=11
  Bus Creator1 : BusCreator  Inputs=8
  Bus Selector : BusSelector  OutputSignals=FIU_SetCH1,FIU_SetCH2,FIU_SetCH3,FIU_SetCH4,FIU_SetCH5,FIU_SetCH6,FIU_SetCH7,FIU_SetCH8
  FIU_CH1 : Subsystem
  FIU_CH2 : Subsystem
  FIU_CH3 : Subsystem
  FIU_CH4 : Subsystem
  FIU_CH5 : Subsystem
  FIU_CH6 : Subsystem
  FIU_CH7 : Subsystem
  FIU_CH8 : Subsystem
  FIU_MsgSend : Subsystem
  YS4008_M_Ctrl_Trigger : Subsystem
  Output : Outport
  wires:
  Bus Creator/1 -> FIU_MsgSend/1(YS4008_M)  "YS4008_M"
  YS4008_M_Ctrl_Trigger/1(YS4008_M_CtrlTrigger) -> FIU_MsgSend/Enable  "Trigger"
  FIU_CH1/1(CH1_Out) -> Bus Creator/2  "CH1_Out"
  FIU_CH2/1(CH2_Out) -> Bus Creator/3  "CH2_Out"
  FIU_CH3/1(CH3_Out) -> Bus Creator/4  "CH3_Out"
  FIU_CH4/1(CH4_Out) -> Bus Creator/5  "CH4_Out"
  FIU_CH5/1(CH5_Out) -> Bus Creator/6  "CH5_Out"
  FIU_CH6/1(CH6_Out) -> Bus Creator/7  "CH6_Out"
  FIU_CH7/1(CH7_Out) -> Bus Creator/8  "CH7_Out"
  FIU_CH8/1(CH8_Out) -> Bus Creator/9  "CH8_Out"
  PassWord/1 -> Bus Creator/1  "PassWord"
  FIU_SetCH1/1 -> Bus Creator1/1  "FIU_SetCH1"
  FIU_SetCH2/1 -> Bus Creator1/2  "FIU_SetCH2"
  FIU_SetCH3/1 -> Bus Creator1/3  "FIU_SetCH3"
  FIU_SetCH7/1 -> Bus Creator1/7  "FIU_SetCH7"
  FIU_SetCH8/1 -> Bus Creator1/8  "FIU_SetCH8"
  FIU_SetCH4/1 -> Bus Creator1/4  "FIU_SetCH4"
  FIU_SetCH5/1 -> Bus Creator1/5  "FIU_SetCH5"
  FIU_SetCH6/1 -> Bus Creator1/6  "FIU_SetCH6"
  Bus Creator1/1 -> [FIU_Set], Bus Selector/1
  [FIU_Set] -> YS4008_M_Ctrl_Trigger/1(YS4008_M)
  Bus Selector/1 -> FIU_CH1/1(FIU_SetCH1)  "<FIU_SetCH1>"
  Bus Selector/2 -> FIU_CH2/1(FIU_SetCH2)  "<FIU_SetCH2>"
  Bus Selector/3 -> FIU_CH3/1(FIU_SetCH3)  "<FIU_SetCH3>"
  Bus Selector/4 -> FIU_CH4/1(FIU_SetCH4)  "<FIU_SetCH4>"
  Bus Selector/5 -> FIU_CH5/1(FIU_SetCH5)  "<FIU_SetCH5>"
  Bus Selector/6 -> FIU_CH6/1(FIU_SetCH6)  "<FIU_SetCH6>"
  Bus Selector/7 -> FIU_CH7/1(FIU_SetCH7)  "<FIU_SetCH7>"
  Bus Selector/8 -> FIU_CH8/1(FIU_SetCH8)  "<FIU_SetCH8>"
  Rack/1 -> Bus Creator/10  "Rack"
  Slot/1 -> Bus Creator/11  "Slot"
  FIU_MsgSend/1(Output) -> Output/1

== system EHB_speedgoat_R2020a_V1/保留/YS4008/YS4008_M_5/YS4008_M ==
  PassWord : Inport
  FIU_SetCH1 : Inport  Port=2
  FIU_SetCH2 : Inport  Port=3
  FIU_SetCH3 : Inport  Port=4
  FIU_SetCH4 : Inport  Port=5
  FIU_SetCH5 : Inport  Port=6
  FIU_SetCH6 : Inport  Port=7
  FIU_SetCH7 : Inport  Port=8
  FIU_SetCH8 : Inport  Port=9
  Rack : Inport  Port=10
  Slot : Inport  Port=11
  Bus Creator : BusCreator  Inputs=11
  Bus Creator1 : BusCreator  Inputs=8
  Bus Selector : BusSelector  OutputSignals=FIU_SetCH1,FIU_SetCH2,FIU_SetCH3,FIU_SetCH4,FIU_SetCH5,FIU_SetCH6,FIU_SetCH7,FIU_SetCH8
  FIU_CH1 : Subsystem
  FIU_CH2 : Subsystem
  FIU_CH3 : Subsystem
  FIU_CH4 : Subsystem
  FIU_CH5 : Subsystem
  FIU_CH6 : Subsystem
  FIU_CH7 : Subsystem
  FIU_CH8 : Subsystem
  FIU_MsgSend : Subsystem
  YS4008_M_Ctrl_Trigger : Subsystem
  Output : Outport
  wires:
  Bus Creator/1 -> FIU_MsgSend/1(YS4008_M)  "YS4008_M"
  YS4008_M_Ctrl_Trigger/1(YS4008_M_CtrlTrigger) -> FIU_MsgSend/Enable  "Trigger"
  FIU_CH1/1(CH1_Out) -> Bus Creator/2  "CH1_Out"
  FIU_CH2/1(CH2_Out) -> Bus Creator/3  "CH2_Out"
  FIU_CH3/1(CH3_Out) -> Bus Creator/4  "CH3_Out"
  FIU_CH4/1(CH4_Out) -> Bus Creator/5  "CH4_Out"
  FIU_CH5/1(CH5_Out) -> Bus Creator/6  "CH5_Out"
  FIU_CH6/1(CH6_Out) -> Bus Creator/7  "CH6_Out"
  FIU_CH7/1(CH7_Out) -> Bus Creator/8  "CH7_Out"
  FIU_CH8/1(CH8_Out) -> Bus Creator/9  "CH8_Out"
  PassWord/1 -> Bus Creator/1  "PassWord"
  FIU_SetCH1/1 -> Bus Creator1/1  "FIU_SetCH1"
  FIU_SetCH2/1 -> Bus Creator1/2  "FIU_SetCH2"
  FIU_SetCH3/1 -> Bus Creator1/3  "FIU_SetCH3"
  FIU_SetCH7/1 -> Bus Creator1/7  "FIU_SetCH7"
  FIU_SetCH8/1 -> Bus Creator1/8  "FIU_SetCH8"
  FIU_SetCH4/1 -> Bus Creator1/4  "FIU_SetCH4"
  FIU_SetCH5/1 -> Bus Creator1/5  "FIU_SetCH5"
  FIU_SetCH6/1 -> Bus Creator1/6  "FIU_SetCH6"
  Bus Creator1/1 -> [FIU_Set], Bus Selector/1
  [FIU_Set] -> YS4008_M_Ctrl_Trigger/1(YS4008_M)
  Bus Selector/1 -> FIU_CH1/1(FIU_SetCH1)  "<FIU_SetCH1>"
  Bus Selector/2 -> FIU_CH2/1(FIU_SetCH2)  "<FIU_SetCH2>"
  Bus Selector/3 -> FIU_CH3/1(FIU_SetCH3)  "<FIU_SetCH3>"
  Bus Selector/4 -> FIU_CH4/1(FIU_SetCH4)  "<FIU_SetCH4>"
  Bus Selector/5 -> FIU_CH5/1(FIU_SetCH5)  "<FIU_SetCH5>"
  Bus Selector/6 -> FIU_CH6/1(FIU_SetCH6)  "<FIU_SetCH6>"
  Bus Selector/7 -> FIU_CH7/1(FIU_SetCH7)  "<FIU_SetCH7>"
  Bus Selector/8 -> FIU_CH8/1(FIU_SetCH8)  "<FIU_SetCH8>"
  Rack/1 -> Bus Creator/10  "Rack"
  Slot/1 -> Bus Creator/11  "Slot"
  FIU_MsgSend/1(Output) -> Output/1

== system EHB_speedgoat_R2020a_V1/保留/YS4008/YS4008_M_6/YS4008_M ==
  PassWord : Inport
  FIU_SetCH1 : Inport  Port=2
  FIU_SetCH2 : Inport  Port=3
  FIU_SetCH3 : Inport  Port=4
  FIU_SetCH4 : Inport  Port=5
  FIU_SetCH5 : Inport  Port=6
  FIU_SetCH6 : Inport  Port=7
  FIU_SetCH7 : Inport  Port=8
  FIU_SetCH8 : Inport  Port=9
  Rack : Inport  Port=10
  Slot : Inport  Port=11
  Bus Creator : BusCreator  Inputs=11
  Bus Creator1 : BusCreator  Inputs=8
  Bus Selector : BusSelector  OutputSignals=FIU_SetCH1,FIU_SetCH2,FIU_SetCH3,FIU_SetCH4,FIU_SetCH5,FIU_SetCH6,FIU_SetCH7,FIU_SetCH8
  FIU_CH1 : Subsystem
  FIU_CH2 : Subsystem
  FIU_CH3 : Subsystem
  FIU_CH4 : Subsystem
  FIU_CH5 : Subsystem
  FIU_CH6 : Subsystem
  FIU_CH7 : Subsystem
  FIU_CH8 : Subsystem
  FIU_MsgSend : Subsystem
  YS4008_M_Ctrl_Trigger : Subsystem
  Output : Outport
  wires:
  Bus Creator/1 -> FIU_MsgSend/1(YS4008_M)  "YS4008_M"
  YS4008_M_Ctrl_Trigger/1(YS4008_M_CtrlTrigger) -> FIU_MsgSend/Enable  "Trigger"
  FIU_CH1/1(CH1_Out) -> Bus Creator/2  "CH1_Out"
  FIU_CH2/1(CH2_Out) -> Bus Creator/3  "CH2_Out"
  FIU_CH3/1(CH3_Out) -> Bus Creator/4  "CH3_Out"
  FIU_CH4/1(CH4_Out) -> Bus Creator/5  "CH4_Out"
  FIU_CH5/1(CH5_Out) -> Bus Creator/6  "CH5_Out"
  FIU_CH6/1(CH6_Out) -> Bus Creator/7  "CH6_Out"
  FIU_CH7/1(CH7_Out) -> Bus Creator/8  "CH7_Out"
  FIU_CH8/1(CH8_Out) -> Bus Creator/9  "CH8_Out"
  PassWord/1 -> Bus Creator/1  "PassWord"
  FIU_SetCH1/1 -> Bus Creator1/1  "FIU_SetCH1"
  FIU_SetCH2/1 -> Bus Creator1/2  "FIU_SetCH2"
  FIU_SetCH3/1 -> Bus Creator1/3  "FIU_SetCH3"
  FIU_SetCH7/1 -> Bus Creator1/7  "FIU_SetCH7"
  FIU_SetCH8/1 -> Bus Creator1/8  "FIU_SetCH8"
  FIU_SetCH4/1 -> Bus Creator1/4  "FIU_SetCH4"
  FIU_SetCH5/1 -> Bus Creator1/5  "FIU_SetCH5"
  FIU_SetCH6/1 -> Bus Creator1/6  "FIU_SetCH6"
  Bus Creator1/1 -> [FIU_Set], Bus Selector/1
  [FIU_Set] -> YS4008_M_Ctrl_Trigger/1(YS4008_M)
  Bus Selector/1 -> FIU_CH1/1(FIU_SetCH1)  "<FIU_SetCH1>"
  Bus Selector/2 -> FIU_CH2/1(FIU_SetCH2)  "<FIU_SetCH2>"
  Bus Selector/3 -> FIU_CH3/1(FIU_SetCH3)  "<FIU_SetCH3>"
  Bus Selector/4 -> FIU_CH4/1(FIU_SetCH4)  "<FIU_SetCH4>"
  Bus Selector/5 -> FIU_CH5/1(FIU_SetCH5)  "<FIU_SetCH5>"
  Bus Selector/6 -> FIU_CH6/1(FIU_SetCH6)  "<FIU_SetCH6>"
  Bus Selector/7 -> FIU_CH7/1(FIU_SetCH7)  "<FIU_SetCH7>"
  Bus Selector/8 -> FIU_CH8/1(FIU_SetCH8)  "<FIU_SetCH8>"
  Rack/1 -> Bus Creator/10  "Rack"
  Slot/1 -> Bus Creator/11  "Slot"
  FIU_MsgSend/1(Output) -> Output/1

== system EHB_speedgoat_R2020a_V1/保留/YS7501_M/HVRealy_Set/CANDataPack_ToUDP ==
  In1 : Inport
  "Bit Packing " : xpcutilitieslib/Bit Packing   MaskBitPatterns={[7],[6],[4 5],[0:3]}  MaskPackDataType=uint8  MaskPackDataSize=[1]
      settings: SourceProductBaseCode=XP
  Bit Slice : hdlsllib/Logic and Bit Operations/Bit Slice  lidx=3  ridx=0
      settings: SourceProductBaseCode=SL
  Bus Selector : BusSelector  OutputSignals=Extended,Length,Remote,ID,Data
  "Byte Packing " : xpcutilitieslib/Byte Packing   MaskPackedDataType=uint8  MaskUnpackedDataTypes={'uint32'}  MaskAlignment=1
  "Byte Reversal " : xpcutilitieslib/Byte Reversal   numInp=1
      settings: SourceProductBaseCode=XP
  Constant1 : Constant  Value=[0 0]
  Data Type Conversion1 : DataTypeConversion  OutDataTypeStr=boolean
  Data Type Conversion2 : DataTypeConversion  OutDataTypeStr=uint8
  Data Type Conversion9 : DataTypeConversion  OutDataTypeStr=boolean
  Mux : Mux  Inputs=3
  Output : Outport
  wires:
  Bus Selector/5 -> Mux/3  "<Data>"
  "Bit Packing "/1 -> Mux/1  "YS5002_PowerSet"
  Bus Selector/2 -> Data Type Conversion2/1  "<Length>"
  Bus Selector/4 -> "Byte Reversal "/1  "<ID>"
  In1/1 -> Bus Selector/1
  Bus Selector/1 -> Data Type Conversion9/1  "<Extended>"
  Bus Selector/3 -> Data Type Conversion1/1  "<Remote>"
  Data Type Conversion9/1 -> "Bit Packing "/1
  "Byte Reversal "/1 -> "Byte Packing "/1
  Bit Slice/1 -> "Bit Packing "/4
  "Byte Packing "/1 -> Mux/2
  Constant1/1 -> "Bit Packing "/3
  Mux/1 -> Output/1
  Data Type Conversion2/1 -> Bit Slice/1
  Data Type Conversion1/1 -> "Bit Packing "/2

== system EHB_speedgoat_R2020a_V1/CAN_Send/CAN Transmit/VCU_Msg/VCU_BrakingRequest_0x120/sigSource1 ==
  InputSignal : Inport
  Constant : Constant  Value=0
  Counter : CanManageLib/Counter  initValue=0  finalValue=15  stepValue=1
  Data Type Conversion : DataTypeConversion
  Multiport Switch : MultiPortSwitch  Inputs=5
  Pulse : DiscretePulseGenerator  Period=10  PulseWidth=5  SampleTime=-1
  Step : Step
  sigType : Constant
  OutputSignal : Outport
  wires:
  Data Type Conversion/1 -> OutputSignal/1
  Multiport Switch/1 -> Data Type Conversion/1
  Pulse/1 -> Multiport Switch/5
  Step/1 -> Multiport Switch/4
  Counter/1 -> Multiport Switch/3
  Constant/1 -> Multiport Switch/6
  InputSignal/1 -> Multiport Switch/2
  sigType/1 -> Multiport Switch/1

== system EHB_speedgoat_R2020a_V1/CAN_Send/CAN Transmit/VCU_Msg/VCU_BrakingRequest_0x120/sigSource2 ==
  InputSignal : Inport
  Constant : Constant  Value=0
  Counter : CanManageLib/Counter  initValue=0  finalValue=15  stepValue=1
  Data Type Conversion : DataTypeConversion
  Multiport Switch : MultiPortSwitch  Inputs=5
  Pulse : DiscretePulseGenerator  Period=10  PulseWidth=5  SampleTime=-1
  Step : Step
  sigType : Constant
  OutputSignal : Outport
  wires:
  Data Type Conversion/1 -> OutputSignal/1
  Multiport Switch/1 -> Data Type Conversion/1
  Pulse/1 -> Multiport Switch/5
  Step/1 -> Multiport Switch/4
  Counter/1 -> Multiport Switch/3
  Constant/1 -> Multiport Switch/6
  InputSignal/1 -> Multiport Switch/2
  sigType/1 -> Multiport Switch/1

== system EHB_speedgoat_R2020a_V1/CAN_Send/CAN Transmit/VCU_Msg/VCU_BrakingRequest_0x120/sigSource3 ==
  InputSignal : Inport
  Constant : Constant  Value=0
  Counter : CanManageLib/Counter  initValue=0  finalValue=15  stepValue=1
  Data Type Conversion : DataTypeConversion
  Multiport Switch : MultiPortSwitch  Inputs=5
  Pulse : DiscretePulseGenerator  Period=10  PulseWidth=5  SampleTime=-1
  Step : Step
  sigType : Constant
  OutputSignal : Outport
  wires:
  Data Type Conversion/1 -> OutputSignal/1
  Multiport Switch/1 -> Data Type Conversion/1
  Pulse/1 -> Multiport Switch/5
  Step/1 -> Multiport Switch/4
  Counter/1 -> Multiport Switch/3
  Constant/1 -> Multiport Switch/6
  InputSignal/1 -> Multiport Switch/2
  sigType/1 -> Multiport Switch/1

== system EHB_speedgoat_R2020a_V1/CAN_Send/Trigger/Trigger_VCU_Msg/Trigger_VCU_BrakingRequest_0x120/Cycle ==
  note: Unsolve
  Add : Sum
  Bias : Bias
  Constant : Constant  Value=EnablePeriod  SampleTime=-1
  Constant1 : Constant  SampleTime=-1
  Delay : Delay  DelayLength=1  ExternalReset=Rising
      settings: InputPortMap=u0,r5
  Delay2 : Delay  DelayLength=1
  Gain : Gain  Gain=1000/(Period)
  MsgLstCnt : Constant  Value=MsgLstCnt  SampleTime=-1
  Multiport Switch : MultiPortSwitch  DataPortOrder=Zero-based contiguous  Inputs=9  DataPortForDefault=Additional data port  zeroidx=on
  Reciprocal : Product  Inputs=/
  Relational Operator : RelationalOperator  Operator=<=  OutDataTypeStr=boolean  RndMeth=Simplest
  Triggered Subsystem1 : Subsystem  TreatAsAtomicUnit=on
  Out1 : Outport  VectorParamsAs1DForOutWhenUnconnected=off
  wires:
  Reciprocal/1 -> Relational Operator/1
  Constant1/1 -> Add/1
  Constant/1 -> Gain/1
  Gain/1 -> Reciprocal/1
  Add/1 -> Relational Operator/2, Delay/1
  Relational Operator/1 -> [SendFlag], Multiport Switch/2, Delay2/1
  Delay/1 -> Add/2
  Delay2/1 -> Delay/2
  Multiport Switch/1 -> Out1/1
  MsgLstCnt/1 -> Bias/1
  Triggered Subsystem1/1(Out1) -> Multiport Switch/4, Multiport Switch/5, Multiport Switch/6, Multiport Switch/7, Multiport Switch/8, Multiport Switch/9, Multiport Switch/10, Multiport Switch/11, Multiport Switch/3
  [MsgLstCnt] -> Triggered Subsystem1/2(MsgLstCnt)
  [SendFlag] -> Triggered Subsystem1/Enable, Triggered Subsystem1/1(SendFlag)
  Bias/1 -> Multiport Switch/1, [MsgLstCnt]

== system EHB_speedgoat_R2020a_V1/CAN_Send/Trigger/Trigger_VCU_Msg/Trigger_VCU_BrakingRequest_0x120/Kick ==
  Delay1 : Delay  DelayLength=1
  KickValue : Constant  SampleTime=-1
  Relational Operator1 : RelationalOperator  Operator=~=  OutDataTypeStr=boolean  RndMeth=Simplest
  Out1 : Outport  VectorParamsAs1DForOutWhenUnconnected=off
  wires:
  KickValue/1 -> Delay1/1, Relational Operator1/1
  Delay1/1 -> Relational Operator1/2
  Relational Operator1/1 -> Out1/1

== system EHB_speedgoat_R2020a_V1/CAN_Send/Trigger/Trigger_VCU_Msg/Trigger_VCU_BrakingRequest_0x120/KickValueChange ==

== system EHB_speedgoat_R2020a_V1/保留/TIF_01/YS4020_M_2/YS4020_M/FIU_CH1 ==
  FIU_SetCH1 : Inport
  "Bit Unpacking " : xpcutilitieslib/Bit Unpacking   SignExtend=on  MaskBitPatterns={[0],[1],[2],[3]}  MaskPackDataType=uint8  MaskPackDataSize=[1]  MaskUnpackDataTypes={'boolean','boolean','boolean','boolean'}  MaskUnpackDataSizes={[1],[1],[1],[1]}
      settings: SourceProductBaseCode=XP
  Bus Creator : BusCreator  Inputs=4
  Protect : Subsystem
  CH1_Out : Outport
  wires:
  Bus Creator/1 -> CH1_Out/1
  "Bit Unpacking "/4 -> Protect/4(Open_In)
  "Bit Unpacking "/3 -> Protect/3(COM_In)
  "Bit Unpacking "/2 -> Protect/2(KL31_In)
  "Bit Unpacking "/1 -> Protect/1(KL30_In)
  Protect/4(Open_Out) -> Bus Creator/4  "Open_Out"
  Protect/1(KL30_Out) -> Bus Creator/1  "KL30_Out"
  Protect/2(KL31_Out) -> Bus Creator/2  "KL31_Out"
  Protect/3(COM_Out) -> Bus Creator/3  "COM_Out"
  FIU_SetCH1/1 -> "Bit Unpacking "/1

== system EHB_speedgoat_R2020a_V1/保留/TIF_01/YS4020_M_2/YS4020_M/FIU_CH10 ==
  FIU_SetCH10 : Inport
  "Bit Unpacking " : xpcutilitieslib/Bit Unpacking   SignExtend=on  MaskBitPatterns={[0],[1],[2],[3]}  MaskPackDataType=uint8  MaskPackDataSize=[1]  MaskUnpackDataTypes={'boolean','boolean','boolean','boolean'}  MaskUnpackDataSizes={[1],[1],[1],[1]}
      settings: SourceProductBaseCode=XP
  Bus Creator : BusCreator  Inputs=4
  Protect : Subsystem
  CH10_Out : Outport
  wires:
  FIU_SetCH10/1 -> "Bit Unpacking "/1
  Protect/3(COM_Out) -> Bus Creator/3  "COM_Out"
  Protect/2(KL31_Out) -> Bus Creator/2  "KL31_Out"
  Protect/1(KL30_Out) -> Bus Creator/1  "KL30_Out"
  Protect/4(Open_Out) -> Bus Creator/4  "Open_Out"
  "Bit Unpacking "/1 -> Protect/1(KL30_In)
  "Bit Unpacking "/2 -> Protect/2(KL31_In)
  "Bit Unpacking "/3 -> Protect/3(COM_In)
  "Bit Unpacking "/4 -> Protect/4(Open_In)
  Bus Creator/1 -> CH10_Out/1

== system EHB_speedgoat_R2020a_V1/保留/TIF_01/YS4020_M_2/YS4020_M/FIU_CH11 ==
  FIU_SetCH1 : Inport
  "Bit Unpacking " : xpcutilitieslib/Bit Unpacking   SignExtend=on  MaskBitPatterns={[0],[1],[2],[3]}  MaskPackDataType=uint8  MaskPackDataSize=[1]  MaskUnpackDataTypes={'boolean','boolean','boolean','boolean'}  MaskUnpackDataSizes={[1],[1],[1],[1]}
      settings: SourceProductBaseCode=XP
  Bus Creator : BusCreator  Inputs=4
  Protect : Subsystem
  CH1_Out : Outport
  wires:
  FIU_SetCH1/1 -> "Bit Unpacking "/1
  Protect/3(COM_Out) -> Bus Creator/3  "COM_Out"
  Protect/2(KL31_Out) -> Bus Creator/2  "KL31_Out"
  Protect/1(KL30_Out) -> Bus Creator/1  "KL30_Out"
  Protect/4(Open_Out) -> Bus Creator/4  "Open_Out"
  "Bit Unpacking "/1 -> Protect/1(KL30_In)
  "Bit Unpacking "/2 -> Protect/2(KL31_In)
  "Bit Unpacking "/3 -> Protect/3(COM_In)
  "Bit Unpacking "/4 -> Protect/4(Open_In)
  Bus Creator/1 -> CH1_Out/1

== system EHB_speedgoat_R2020a_V1/保留/TIF_01/YS4020_M_2/YS4020_M/FIU_CH12 ==
  FIU_SetCH10 : Inport
  "Bit Unpacking " : xpcutilitieslib/Bit Unpacking   SignExtend=on  MaskBitPatterns={[0],[1],[2],[3]}  MaskPackDataType=uint8  MaskPackDataSize=[1]  MaskUnpackDataTypes={'boolean','boolean','boolean','boolean'}  MaskUnpackDataSizes={[1],[1],[1],[1]}
      settings: SourceProductBaseCode=XP
  Bus Creator : BusCreator  Inputs=4
  Protect : Subsystem
  CH10_Out : Outport
  wires:
  Bus Creator/1 -> CH10_Out/1
  "Bit Unpacking "/4 -> Protect/4(Open_In)
  "Bit Unpacking "/3 -> Protect/3(COM_In)
  "Bit Unpacking "/2 -> Protect/2(KL31_In)
  "Bit Unpacking "/1 -> Protect/1(KL30_In)
  Protect/4(Open_Out) -> Bus Creator/4  "Open_Out"
  Protect/1(KL30_Out) -> Bus Creator/1  "KL30_Out"
  Protect/2(KL31_Out) -> Bus Creator/2  "KL31_Out"
  Protect/3(COM_Out) -> Bus Creator/3  "COM_Out"
  FIU_SetCH10/1 -> "Bit Unpacking "/1
